simulink model "task3"  (R2024a)
settings: Solver=VariableStepAuto  StartTime=0.0  StopTime=10.0  MaxStep=0.01  RelTol=1e-3
undefined symbols (not defined in the file): A, A_bar, B, Bf, C, CZ, D, DZ, G, K1, K2, L, w0, x0, xw0_hat, YZ
settings Model: Creator=sizgr  LastModifiedBy=sizgr

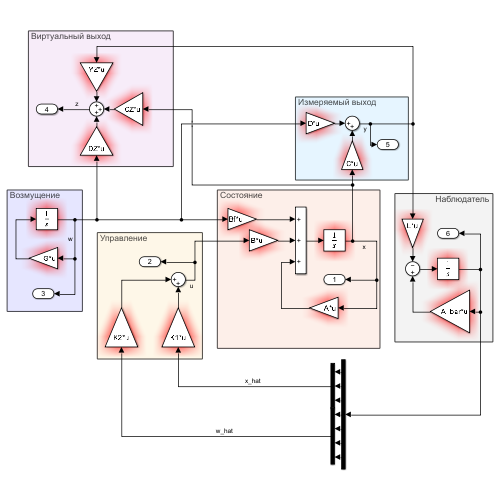
[thumbnail: Simulink's stored preview of the top-level diagram]
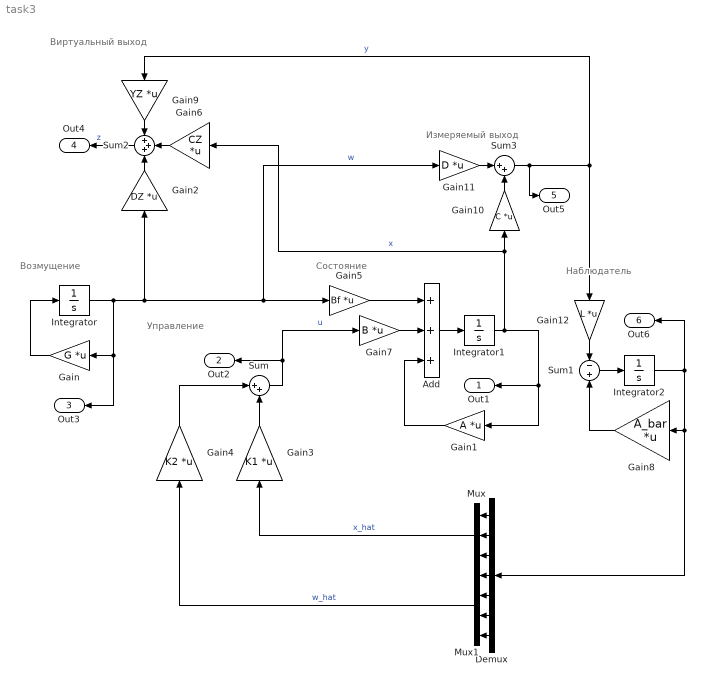
== system task3 ==
  note: Наблюдатель
  note: Измеряемый выход
  note: Состояние
  note: Виртуальный выход
  note: Управление
  note: Возмущение
  Add : Sum  Inputs=+++
  Demux : Demux  Outputs=7
  Gain : Gain  Gain=G  Multiplication=Matrix(K*u)
  Gain1 : Gain  Gain=A  Multiplication=Matrix(K*u)
  Gain10 : Gain  Gain=C  Multiplication=Matrix(K*u)
  Gain11 : Gain  Gain=D  Multiplication=Matrix(K*u)
  Gain12 : Gain  Gain=L  Multiplication=Matrix(K*u)
  Gain2 : Gain  Gain=DZ  Multiplication=Matrix(K*u)
  Gain3 : Gain  Gain=K1  Multiplication=Matrix(K*u)
  Gain4 : Gain  Gain=K2  Multiplication=Matrix(K*u)
  Gain5 : Gain  Gain=Bf  Multiplication=Matrix(K*u)
  Gain6 : Gain  Gain=CZ  Multiplication=Matrix(K*u)
  Gain7 : Gain  Gain=B  Multiplication=Matrix(K*u)
  Gain8 : Gain  Gain=A_bar  Multiplication=Matrix(K*u)
  Gain9 : Gain  Gain=YZ  Multiplication=Matrix(K*u)
  Integrator : Integrator  InitialCondition=w0
  Integrator1 : Integrator  InitialCondition=x0
  Integrator2 : Integrator  InitialCondition=xw0_hat
  Mux : Mux  Inputs=3
  Mux1 : Mux
  Sum : Sum  Inputs=|++
  Sum1 : Sum  Inputs=-|+
  Sum2 : Sum  Inputs=+++
  Sum3 : Sum  Inputs=|++
  Out1 : Outport
  Out2 : Outport  Port=2
  Out3 : Outport  Port=3
  Out4 : Outport  Port=4
  Out5 : Outport  Port=5
  Out6 : Outport  Port=6
  wires:
  Integrator/1 -> Out3/1, Gain/1, Gain11/1, Gain5/1, Gain2/1  "w"
  Gain/1 -> Integrator/1
  Integrator1/1 -> Gain1/1, Out1/1, Gain6/1, Gain10/1  "x"
  Gain1/1 -> Add/3
  Add/1 -> Integrator1/1
  Gain4/1 -> Sum/1
  Gain3/1 -> Sum/2
  Sum/1 -> Gain7/1, Out2/1  "u"
  Gain5/1 -> Add/1
  Sum2/1 -> Out4/1  "z"
  Gain7/1 -> Add/2
  Sum1/1 -> Integrator2/1
  Integrator2/1 -> Out6/1, Demux/1, Gain8/1
  Gain8/1 -> Sum1/2
  Sum3/1 -> Gain9/1, Gain12/1, Out5/1  "y"
  Gain11/1 -> Sum3/1
  Gain10/1 -> Sum3/2
  Gain12/1 -> Sum1/1
  Demux/1 -> Mux/1
  Demux/2 -> Mux/2
  Demux/3 -> Mux/3
  Demux/4 -> Mux1/1
  Demux/5 -> Mux1/2
  Demux/6 -> Mux1/3
  Demux/7 -> Mux1/4
  Mux/1 -> Gain3/1  "x_hat"
  Mux1/1 -> Gain4/1  "w_hat"
  Gain6/1 -> Sum2/2
  Gain2/1 -> Sum2/3
  Gain9/1 -> Sum2/1
